simulink model "mod_feedback"  (R2024b)
settings: Solver=VariableStepAuto  StartTime=0.0  StopTime=10.0  RelTol=1e-3
values from neighbouring files (symbols this model uses):
  Kc = 4    [es_reti_compensazione.m]
settings Model: Creator=jacoposini  LastModifiedBy=jacoposini

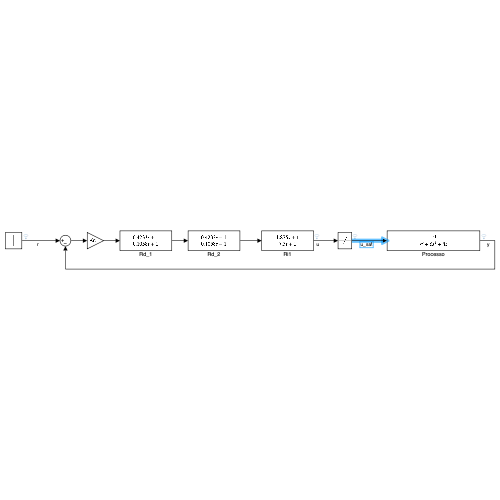
[thumbnail: Simulink's stored preview of the top-level diagram]
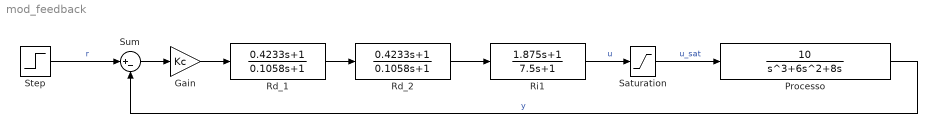
== system mod_feedback ==
  Gain : Gain  Gain=Kc
  Processo : TransferFcn  Numerator=[10]  Denominator=[1 6 8 0]
  Rd_1 : TransferFcn  Numerator=[0.4233 1]  Denominator=[0.1058 1]
  Rd_2 : TransferFcn  Numerator=[0.4233 1]  Denominator=[0.1058 1]
  Ri1 : TransferFcn  Numerator=[1.875 1]  Denominator=[7.5 1]
  Saturation : Saturate  UpperLimit=20  LowerLimit=-20
  Step : Step  SampleTime=0
  Sum : Sum  Inputs=|+-
  wires:
  Sum/1 -> Gain/1
  Processo/1 -> Sum/2  "y"
  Step/1 -> Sum/1  "r"
  Gain/1 -> Rd_1/1
  Rd_1/1 -> Rd_2/1
  Rd_2/1 -> Ri1/1
  Saturation/1 -> Processo/1  "u_sat"
  Ri1/1 -> Saturation/1  "u"
